simulink model "Ejercicio2"  (R2025a)
settings: Solver=ode8  StartTime=0.0  StopTime=10  FixedStep=1e-4  RelTol=1e-3
values from neighbouring files (symbols this model uses):
  G_array = cat(3, G_cell{:})    [Constantes1.m]    (also in Constantes2.m)
  K_array = cat(3, K_cell{:})    [Constantes1.m]    (also in Constantes2.m)
  P_array = cat(3, P_cell{:})    [Constantes1.m]    (also in Constantes2.m)
settings Model: Creator=440G5  LastModifiedBy=440G5

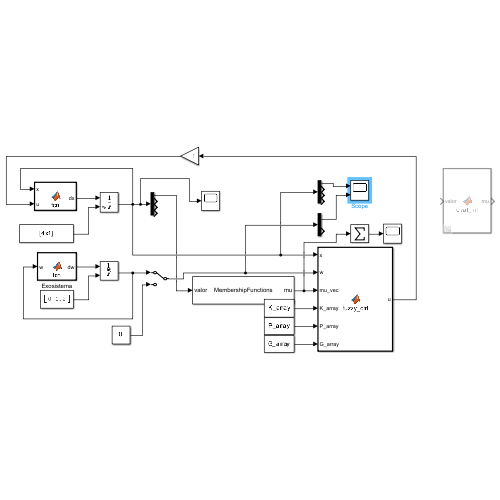
[thumbnail: Simulink's stored preview of the top-level diagram]
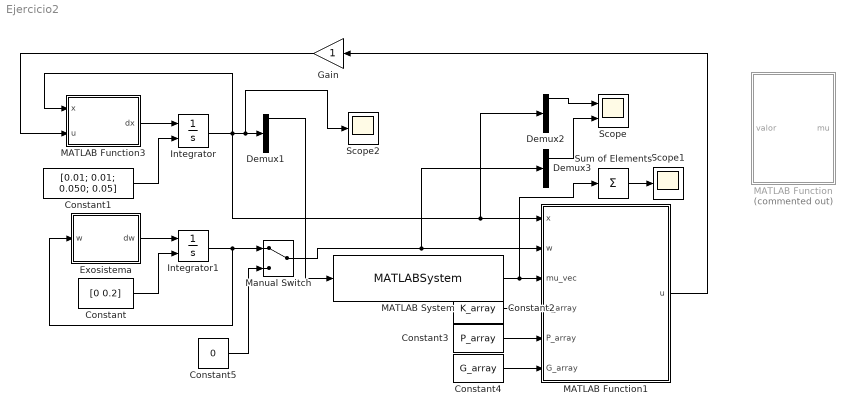
== system Ejercicio2 ==
  Constant : Constant  Value=[0 0.2]
  Constant1 : Constant  Value=[0.01; 0.01; 0.050; 0.05]
  Constant2 : Constant  Value=K_array
  Constant3 : Constant  Value=P_array
  Constant4 : Constant  Value=G_array
  Constant5 : Constant  Value=0
  Demux1 : Demux
  Demux2 : Demux
  Demux3 : Demux  Outputs=2
  Exosistema : MATLAB Function  TreatAsAtomicUnit=on
  Gain : Gain
  Integrator : Integrator  InitialConditionSource=external
  Integrator1 : Integrator  InitialConditionSource=external
  MATLAB Function : MATLAB Function  Commented=on  TreatAsAtomicUnit=on
  MATLAB Function1 : MATLAB Function  TreatAsAtomicUnit=on
  MATLAB Function3 : MATLAB Function  TreatAsAtomicUnit=on
  MATLAB System : MATLABSystem  System=MembershipFunctions  N=20  Range=[ -15, 15 ]  InputIsRadians=true  SimulateUsing=Interpreted execution
      mask Type: MembershipFunctions
  Manual Switch : ManualSwitch
  Scope : Scope  NumInputPorts=2
      settings: ActiveDisplayYMinimum=-1.0191728417035857  ActiveDisplayYMaximum=1.6224108807295476
  Scope1 : Scope
      settings: ActiveDisplayYMinimum=0.99999999999999978  ActiveDisplayYMaximum=1
  Scope2 : Scope
      settings: ActiveDisplayYMinimum=-1045.5602210262018  ActiveDisplayYMaximum=830.04177518311019  DataLoggingVariableName=ScopeData2
  Sum of Elements : Sum  Inputs=+
  wires:
  MATLAB System/1 -> Sum of Elements/1, MATLAB Function1/3(mu_vec)
  Integrator/1 -> Scope2/1, Demux1/1, MATLAB Function1/1(x), Demux2/1, MATLAB Function3/1(x)
  MATLAB Function3/1(dx) -> Integrator/1
  Constant1/1 -> Integrator/2
  Exosistema/1(dw) -> Integrator1/1
  Constant/1 -> Integrator1/2
  Integrator1/1 -> Manual Switch/1, Exosistema/1(w)
  Constant2/1 -> MATLAB Function1/4(K_array)
  Constant3/1 -> MATLAB Function1/5(P_array)
  Constant4/1 -> MATLAB Function1/6(G_array)
  Sum of Elements/1 -> Scope1/1
  MATLAB Function1/1(u) -> Gain/1
  Demux3/1 -> Scope/2
  Manual Switch/1 -> Demux3/1, MATLAB Function1/2(w)
  Constant5/1 -> Manual Switch/2
  Gain/1 -> MATLAB Function3/2(u)
  Demux2/1 -> Scope/1
  Demux1/1 -> MATLAB System/1

== matlab function Ejercicio2/MATLAB Function1 ==
  data: x input; u output; w input; mu_vec input; K_array input; P_array input; G_array input
function u = fuzzy_ctrl(x, w, mu_vec, K_array, P_array, G_array)
% Control difuso Takagi–Sugeno + Regulación Lineal (Francis)
% x: 4x1, w: 2x1, mu_vec: 1xN, K_array: 1x4xN, P_array: 4x2xN, G_array: 1x2xN

N = numel(mu_vec);
u_num = 0; u_den = 0;

for i = 1:N
    Ki = K_array(:,:,i);   % 1x4
    Pi = P_array(:,:,i);   % 4x2
    Gi = G_array(:,:,i);   % 1x2

    ui = -Ki*x + (Gi - Ki*Pi)*w; % ley local
    u_num = u_num + mu_vec(i)*ui;
    u_den = u_den + mu_vec(i);
end

if u_den > 0
    u = u_num / u_den;
else
    u = 0;
end
end

== matlab function Ejercicio2/MATLAB Function ==
  data: mu output; valor input
function mu = eval_mf(valor)
% Número de funciones de membresía (constante)
N = 5;
rango = [-15 15];

% Inicializar salida con tamaño fijo
mu = zeros(1,N);

rmin = rango(1);
rmax = rango(2);
step = (rmax - rmin) / (N - 1);
centers = rmin:step:rmax;

for i = 1:N
    if i == 1
        if valor <= centers(1)
            mu(i) = 1;
        elseif valor >= centers(2)
            mu(i) = 0;
        else
            mu(i) = (centers(2) - valor) / (centers(2) - centers(1));
        end

    elseif i == N
        if valor >= centers(end)
            mu(i) = 1;
        elseif valor <= centers(end-1)
            mu(i) = 0;
        else
            mu(i) = (valor - centers(end-1)) / (centers(end) - centers(end-1));
        end

    else
        left = centers(i-1);
        mid  = centers(i);
        right = centers(i+1);

        if valor == mid
            mu(i) = 1;
        elseif valor > left && valor < mid
            mu(i) = (valor - left) / (mid - left);
        elseif valor > mid && valor < right
            mu(i) = (right - valor) / (right - mid);
        else
            mu(i) = 0;
        end
    end
end

== matlab function Ejercicio2/Exosistema ==
  data: w input; dw output
function dw = fcn(w)

dw = [0 10; -10 0]*w;

== matlab function Ejercicio2/MATLAB Function3 ==
  data: x input; u input; dx output
function dx= fcn(x, u)
% Rotary inverted pendulum (Furuta)
% State: x = [beta; betadot; gamma; gammadot]
%
% Parameters (set these to your hardware):
g   = 9.81;     % [m/s^2]
m2  = 0.50;     % [kg]   pendulum mass
l1  = 0.12;     % [m]    arm length to pivot
l2  = 0.75;     % [m]    pendulum COM distance from pivot
J   = 0.003;    % [kg*m^2] motor+arm inertia about base axis

% Viscous friction (set to 0 if unknown)
b_beta  = 0.0;  % [N*m*s/rad] at pendulum joint
b_gamma = 0.0;  % [N*m*s/rad] at base (motor) axis

% Motor/electrics (set to your real values)
Kg = 1.0;       % gear ratio
Km = 1.0;       % [N*m/A] (also V*s/rad in SI)
Rm = 1.0;       % [Ohm]
P1 = (Kg*Km)/Rm;
P2 = (Kg*Km)^2/Rm;

% Unpack state
beta   = x(1);
betad  = x(2);
gamma  = x(3); %#ok<NASGU> % (not used explicitly in the model)
gammad = x(4);

% Inertia matrix D(q) with q = [gamma; beta]
d11 = m2*l1^2 + J;
d12 =  m2*l1*l2*cos(beta);
d21 =  d12;
d22 =  m2*l2^2;

% Coriolis/centrífuga term C(q,qd)*qd -> only c12*betad appears
c12 = -m2*l1*l2*sin(beta)*betad;
% Gravity vector G(q) = [0; g2]
g2 = -m2*l2*g*sin(beta);

% Motor torque at base axis (input side): tau1 = P1*u - P2*gammad
%tau1 = P1*u - P2*gammad;
% Usa entrada como torque directo:
tau1 = u;    % <-- en lugar de P1*u - P2*x4

% Optional viscous frictions moved to RHS
% Equation form:
% d11*ddgamma + d12*ddbeta + c12*betad + b_gamma*gammad = tau1
% d21*ddgamma + d22*ddbeta +          b_beta*betad + g2 = 0

rhs1 = tau1 - c12*betad - b_gamma*gammad;
rhs2 = -g2 - b_beta*betad;

% Solve [ddgamma; ddbeta] = inv(D)*[rhs1; rhs2]
Delta   = d11*d22 - d12*d21;

if Delta < 1e-6
    Delta = 1e-6;  % evita explosión numérica mientras depuras
end

inv11   =  d22 / Delta;
inv12   = -d12 / Delta;
inv21   = -d21 / Delta;
inv22   =  d11 / Delta;

ddgamma = inv11*rhs1 + inv12*rhs2;
ddbeta  = inv21*rhs1 + inv22*rhs2;

% Assemble state derivative
dx = zeros(4,1);
dx(1) = betad;
dx(2) = ddbeta;
dx(3) = gammad;
dx(4) = ddgamma;

% (Optional) measured output if you need it:
y = beta;           % angle of pendulum
y2 = beta + gamma;  % auxiliary output often used in papers

end
